simulink library "command_generation"  (R2016b)
settings: Solver=VariableStepAuto  StartTime=0.0  StopTime=10.0  RelTol=1e-3
libraries: momentum_dump_lib x1, pd_control_lib x1, bdot_controller_lib x1, command_processing x1
settings Model: Creator=taylorreynolds  LastModifiedBy=Taylor

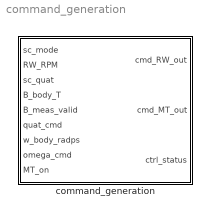
== system command_generation ==
  command_generation : Subsystem

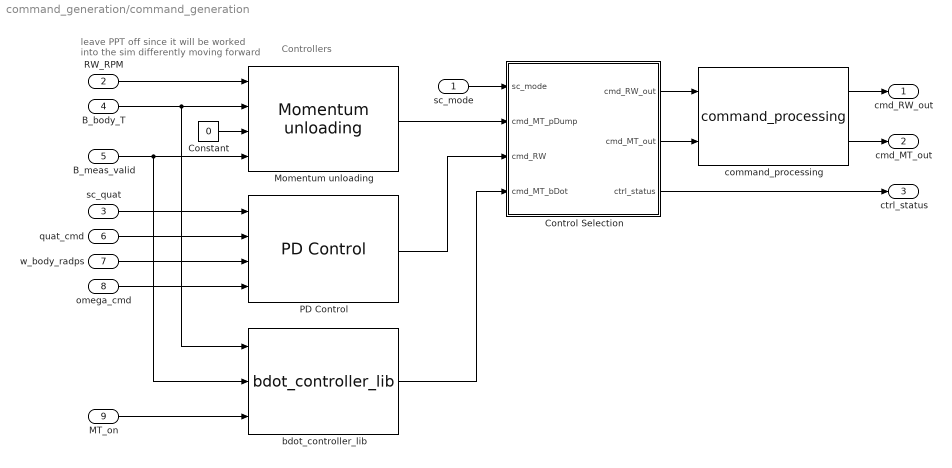
== system command_generation/command_generation ==
  note: Controllers
  note: leave PPT off since it will be
      | worked into the sim differently
      | moving forward
  sc_mode : Inport
  RW_RPM : Inport  Port=2
  sc_quat : Inport  Port=3
  B_body_T : Inport  Port=4
  B_meas_valid : Inport  Port=5
  quat_cmd : Inport  Port=6
  w_body_radps : Inport  Port=7
  omega_cmd : Inport  Port=8
  MT_on : Inport  Port=9
  Constant : Constant  Value=0
  Control Selection : Subsystem
  Momentum unloading : momentum_dump_lib/Momentum unloading
  PD Control : pd_control_lib/PD Control
  bdot_controller_lib : bdot_controller_lib/bdot_controller_lib
  command_processing : command_processing/command_processing
  cmd_RW_out : Outport
  cmd_MT_out : Outport  Port=2
  ctrl_status : Outport  Port=3
  wires:
  RW_RPM/1 -> Momentum unloading/1
  B_body_T/1 -> bdot_controller_lib/1, Momentum unloading/2
  B_meas_valid/1 -> Momentum unloading/4, bdot_controller_lib/2
  command_processing/2 -> cmd_MT_out/1
  command_processing/1 -> cmd_RW_out/1
  Control Selection/1(cmd_RW_out) -> command_processing/1
  Control Selection/2("cmd_MT_out ") -> command_processing/2
  Control Selection/3(ctrl_status) -> ctrl_status/1
  sc_mode/1 -> Control Selection/1(sc_mode)
  Momentum unloading/1 -> Control Selection/2(cmd_MT_pDump)
  PD Control/1 -> Control Selection/3(cmd_RW)
  quat_cmd/1 -> PD Control/2
  sc_quat/1 -> PD Control/1
  w_body_radps/1 -> PD Control/3
  omega_cmd/1 -> PD Control/4
  Constant/1 -> Momentum unloading/3
  MT_on/1 -> bdot_controller_lib/3
  bdot_controller_lib/1 -> Control Selection/4(cmd_MT_bDot)

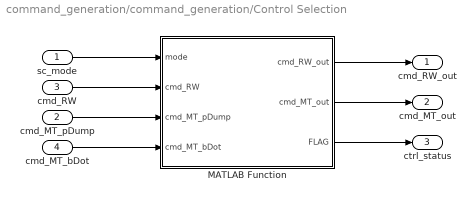
== system command_generation/command_generation/Control Selection ==
  sc_mode : Inport
  cmd_MT_pDump : Inport  Port=2
  cmd_RW : Inport  Port=3
  cmd_MT_bDot : Inport  Port=4
  MATLAB Function : MATLAB Function  TreatAsAtomicUnit=on
  cmd_RW_out : Outport
  "cmd_MT_out " : Outport  Port=2
  ctrl_status : Outport  Port=3
  wires:
  sc_mode/1 -> MATLAB Function/1(mode)
  cmd_RW/1 -> MATLAB Function/2(cmd_RW)
  cmd_MT_pDump/1 -> MATLAB Function/3(cmd_MT_pDump)
  MATLAB Function/1(cmd_RW_out) -> cmd_RW_out/1
  MATLAB Function/2(cmd_MT_out) -> "cmd_MT_out "/1
  MATLAB Function/3(FLAG) -> ctrl_status/1
  cmd_MT_bDot/1 -> MATLAB Function/4(cmd_MT_bDot)

== matlab function command_generation/Control Selection/MATLAB Function ==
  data: mode input; cmd_RW_out output; cmd_RW input; cmd_MT_pDump input; cmd_MT_out output; FLAG output; cmd_MT_bDot input
 function [cmd_RW_out,cmd_MT_out,FLAG] = fcn(mode,cmd_RW,cmd_MT_pDump,cmd_MT_bDot)
% Control Selection Logic
%
% Selects which command gets passed to the actuators based on the mode
% provided by upstream mode selection. Current modes are:
%   mode_logic.bdot             = 1;
%   mode_logic.desat_eclipse    = 2;
%   mode_logic.point            = 3;
%       point.velocity          = 31;
%       point.ground            = 32;
%   mode_logic.low_power        = 4;
%
% FLAG output can be used to make sure the control output matches up with
% what is being commanded, before commands are passed to actuators. FLAG
% should match mode, unless something is wrong.
%
% RAIN-SAT: T. Reynolds 7.7.18

FLAG    = 1;

if( mode == 1 )
    cmd_RW_out      = zeros(3,1);
    cmd_MT_out      = cmd_MT_bDot;
elseif( mode == 2 )
    cmd_RW_out      = cmd_RW;
    cmd_MT_out      = cmd_MT_pDump;
elseif( mode == 31 || mode == 32 || mode == 33 )
    cmd_RW_out      = cmd_RW;
    cmd_MT_out      = cmd_MT_pDump;
elseif( mode == 4 )
    cmd_RW_out      = zeros(3,1);
    cmd_MT_out      = zeros(3,1);
else
    FLAG = -1;
    cmd_RW_out      = zeros(3,1);
    cmd_MT_out      = zeros(3,1);
end
